simulink model "SADproject"  (R2022b)
settings: Solver=ode5  StartTime=0.0  StopTime=Tsc  FixedStep=0.1  MaxStep=0.1  RelTol=1e-6
values from neighbouring files (symbols this model uses):
  a = R_E+altittude    [SCparameters.m]
  A_iw = [-1  1  1 -1 ... (first row only)    [SCparameters.m]
  A_lin = [     zeros(3)       ,        eye(3) ... (first row only)    [SCparameters.m]
  Ai = [A1 A2 A3 A4 A5 A6 A7 A8 A9 A10]    [SCparameters.m]
  Ai_LN = [1    0      0 ... (first row only)    [SCparameters.m]
  ARW_gyro = 0.15    [SCparameters.m]
  B_lin = [zeros(3); diag(1./diag(J))]    [SCparameters.m]
  bias_gyro = 0.3    [SCparameters.m]
  C_lin = [eye(3), zeros(3)]    [SCparameters.m]
  c_m = (R_E^3*H0)/a^3    [SCparameters.m]
  err_HS = 0.1    [SCparameters.m]
  err_SS = 0.1    [SCparameters.m]
  Fe_E = 117    [SCparameters.m]
  Fe_reflected = 500    [SCparameters.m]
  Fe_Sun = astroConstants(31)    [SCparameters.m]
  i = acos(-(a/12352)^(7/2))    [SCparameters.m]
  i_E = astroConstants(8)    [SCparameters.m]
  i_m = deg2rad(11.5)    [SCparameters.m]
  J = I_body + I_panel1 + I_panel2    [SCparameters.m]
  L = place(A_lin',C_lin',CLP)'    [SCparameters.m]
  m = [0.01 0.05 0.01]'    [SCparameters.m]
  maxL_iw = 6*1e-3    (= 0.006)    [SCparameters.m]
  maxT_iw = 0.1*1e-3    (= 0.0001)    [SCparameters.m]
  n = sqrt(muE/a^3)    [SCparameters.m]
  N_Bi = [n1; n2; n3; n4; n5; n6; n7; n8; n9; n10]    [SCparameters.m]
  n_Sun = 2*pi/T_E    (= 1.99098857148e-07)    [SCparameters.m]
  om0 = [1 1 1]'    [SCparameters.m]
  om_E = 7.292*1e-5    (= 7.292e-05)    [SCparameters.m]
  pinvA_iw = [-1 -1  1 ... (first row only)    [SCparameters.m]
  R_t = [R_t1; R_t2]    [SCparameters.m]
  Ri = [b0; b0; b0; b0; b0; b0; b1; b1; b2; b2]    [SCparameters.m]
  T = 0.005    [SCparameters.m]
undefined symbols (not defined in the file or in its folder): K
libraries: vrlib x13, matrix_library x8, dspinverses x2, simulink_extras x2, sharedutil x2, aerolibutil x1
settings Model: Creator=franc  LastModifiedBy=franc
settings SolverCC: AlgebraicLoopSolver=TrustRegion
settings DebuggingCC: UnconnectedInputMsg=warning  UnconnectedOutputMsg=warning  UnconnectedLineMsg=warning  SFMachineParentedDataDiag=warning
settings ModelReferenceCC: EnableRefExpFcnMdlSchedulingChecks=on

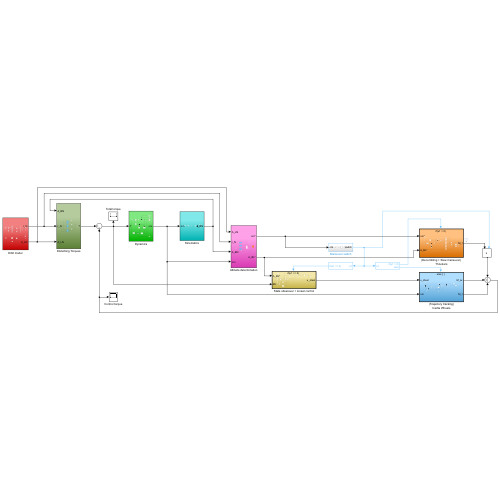
[thumbnail: Simulink's stored preview of the top-level diagram]
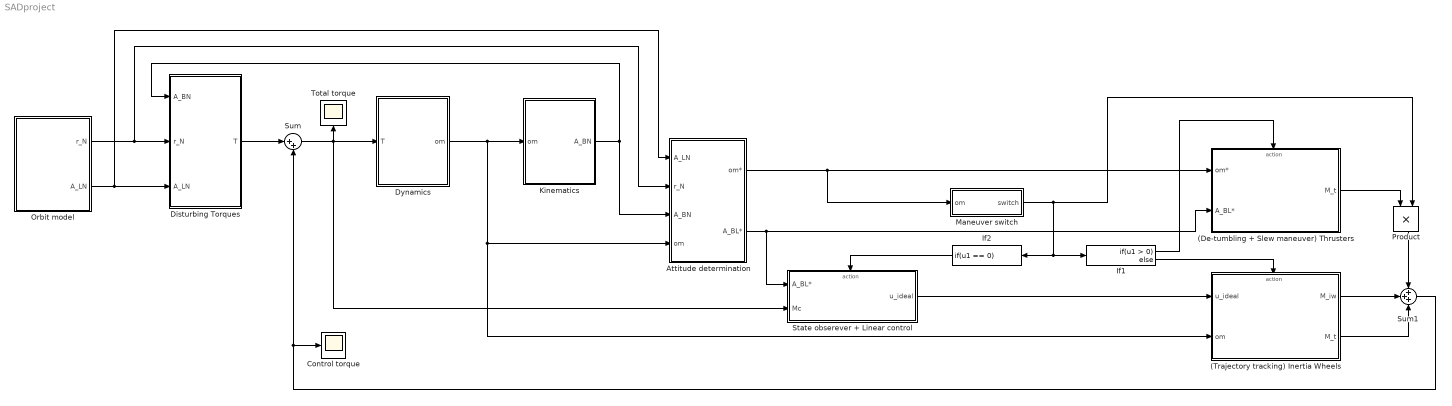
== system SADproject ==
  (De-tumbling + Slew maneuver) Thrusters : Subsystem  TreatAsAtomicUnit=on
  (Trajectory tracking) Inertia Wheels : Subsystem  TreatAsAtomicUnit=on
  Attitude determination : Subsystem
  Control torque : Scope
  Disturbing Torques : Subsystem
  Dynamics : Subsystem
  If1 : If
  If2 : If  IfExpression=u1 == 0  ShowElse=off
  Kinematics : Subsystem
  Maneuver switch : Subsystem
  "Orbit model " : Subsystem
  Product : Product
  State obserever + Linear control : Subsystem
  Sum : Sum  Inputs=|++
  Sum1 : Sum  Inputs=+++
  Total torque : Scope
  wires:
  (De-tumbling + Slew maneuver) Thrusters/1(M_t) -> Product/1
  (Trajectory tracking) Inertia Wheels/1(M_iw) -> Sum1/2
  Product/1 -> Sum1/1
  (Trajectory tracking) Inertia Wheels/2(M_t) -> Sum1/3
  Sum1/1 -> Sum/2, Control torque/1
  State obserever + Linear control/1(u_ideal) -> (Trajectory tracking) Inertia Wheels/1(u_ideal)
  Sum/1 -> State obserever + Linear control/2(Mc), Dynamics/1(T), Total torque/1
  Maneuver switch/1(switch) -> If2/1, If1/1, Product/2
  If1/1 -> (De-tumbling + Slew maneuver) Thrusters/Action
  If1/2 -> (Trajectory tracking) Inertia Wheels/Action
  If2/1 -> State obserever + Linear control/Action
  Dynamics/1(om) -> Kinematics/1(om), (Trajectory tracking) Inertia Wheels/2(om), Attitude determination/4(om)
  Attitude determination/2(A_BL*) -> State obserever + Linear control/1(A_BL*), (De-tumbling + Slew maneuver) Thrusters/2(A_BL*)
  Attitude determination/1(om*) -> (De-tumbling + Slew maneuver) Thrusters/1(om*), Maneuver switch/1(om)
  Kinematics/1(A_BN) -> Attitude determination/3(A_BN), Disturbing Torques/1(A_BN)
  "Orbit model "/1(r_N) -> Disturbing Torques/2(r_N), Attitude determination/2(r_N)
  "Orbit model "/2(A_LN) -> Disturbing Torques/3(A_LN), Attitude determination/1(A_LN)
  Disturbing Torques/1(T) -> Sum/1

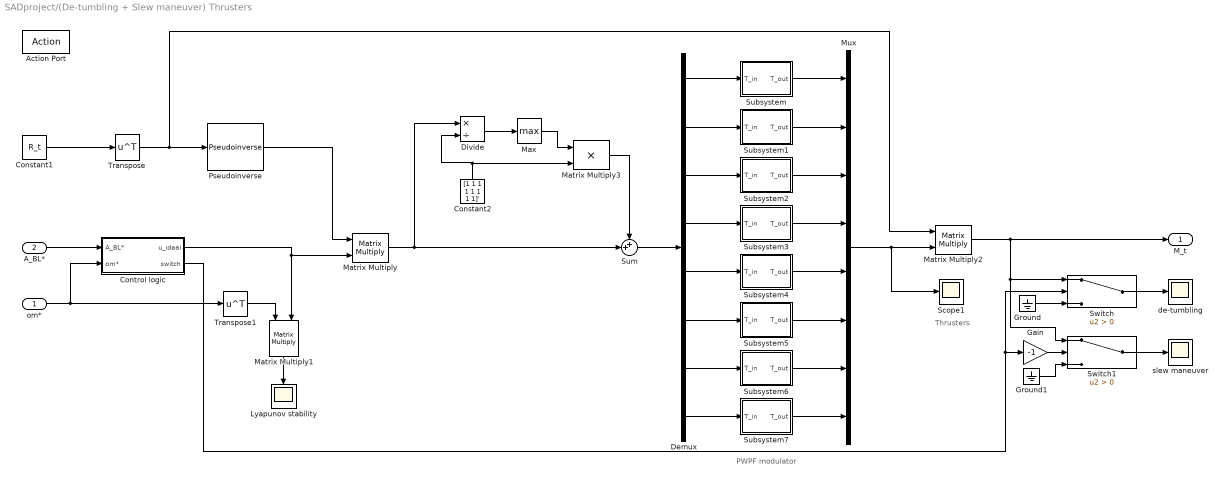
== system SADproject/(De-tumbling + Slew maneuver) Thrusters ==
  note: Thrusters
  note: PWPF modulator
  om* : Inport
  A_BL* : Inport  Port=2
  Action Port : ActionPort  ActionPortLabel=if(u1 > 0)
  Constant1 : Constant  Value=R_t
  Constant2 : Constant  Value=[1 1 1 1 1 1 1 1]'
  Control logic : Subsystem
  Demux : Demux  Outputs=8
  Divide : Product  Inputs=*/
  Gain : Gain  Gain=-1
  Ground : Ground
  Ground1 : Ground
  Lyapunov stability : Scope
  Matrix Multiply : Product  Multiplication=Matrix(*)
  Matrix Multiply1 : Product  Multiplication=Matrix(*)
  Matrix Multiply2 : Product  Multiplication=Matrix(*)
  Matrix Multiply3 : Product
  Max : MinMax  Function=max
  Mux : Mux  Inputs=8
  Pseudoinverse : dspinverses/Pseudoinverse  wanterr=off  SimulateUsing=Interpreted execution
  Scope1 : Scope
  Subsystem : Subsystem
  Subsystem1 : Subsystem
  Subsystem2 : Subsystem
  Subsystem3 : Subsystem
  Subsystem4 : Subsystem
  Subsystem5 : Subsystem
  Subsystem6 : Subsystem
  Subsystem7 : Subsystem
  Sum : Sum  Inputs=++|
  Switch : Switch  Criteria=u2 > Threshold  SaturateOnIntegerOverflow=off  InputSameDT=off
  Switch1 : Switch  Criteria=u2 > Threshold  SaturateOnIntegerOverflow=off  InputSameDT=off
  Transpose : Math  Operator=transpose
  Transpose1 : Math  Operator=transpose
  de-tumbling : Scope
  slew maneuver : Scope
  M_t : Outport
  wires:
  Subsystem1/1(T_out) -> Mux/2
  Demux/8 -> Subsystem7/1(T_in)
  Demux/7 -> Subsystem6/1(T_in)
  Subsystem2/1(T_out) -> Mux/3
  Subsystem7/1(T_out) -> Mux/8
  Demux/4 -> Subsystem3/1(T_in)
  Subsystem3/1(T_out) -> Mux/4
  Demux/6 -> Subsystem5/1(T_in)
  Demux/2 -> Subsystem1/1(T_in)
  Demux/3 -> Subsystem2/1(T_in)
  Constant2/1 -> Matrix Multiply3/2, Divide/2
  Subsystem5/1(T_out) -> Mux/6
  Matrix Multiply1/1 -> Lyapunov stability/1
  Matrix Multiply2/1 -> Switch1/1, Switch/1, M_t/1
  Subsystem/1(T_out) -> Mux/1
  Mux/1 -> Scope1/1, Matrix Multiply2/2
  Matrix Multiply3/1 -> Sum/1
  om*/1 -> Control logic/2(om*), Transpose1/1
  Subsystem6/1(T_out) -> Mux/7
  Pseudoinverse/1 -> Matrix Multiply/1
  Divide/1 -> Max/1
  Matrix Multiply/1 -> Sum/2, Divide/1
  Max/1 -> Matrix Multiply3/1
  Constant1/1 -> Transpose/1
  Transpose/1 -> Matrix Multiply2/1, Pseudoinverse/1
  Demux/1 -> Subsystem/1(T_in)
  Control logic/1(u_ideal) -> Matrix Multiply/2, Matrix Multiply1/2
  Demux/5 -> Subsystem4/1(T_in)
  Sum/1 -> Demux/1
  Subsystem4/1(T_out) -> Mux/5
  Transpose1/1 -> Matrix Multiply1/1
  A_BL*/1 -> Control logic/1(A_BL*)
  Control logic/2(switch) -> Switch/2, Gain/1
  Ground/1 -> Switch/3
  Switch/1 -> de-tumbling/1
  Gain/1 -> Switch1/2
  Ground1/1 -> Switch1/3
  Switch1/1 -> slew maneuver/1

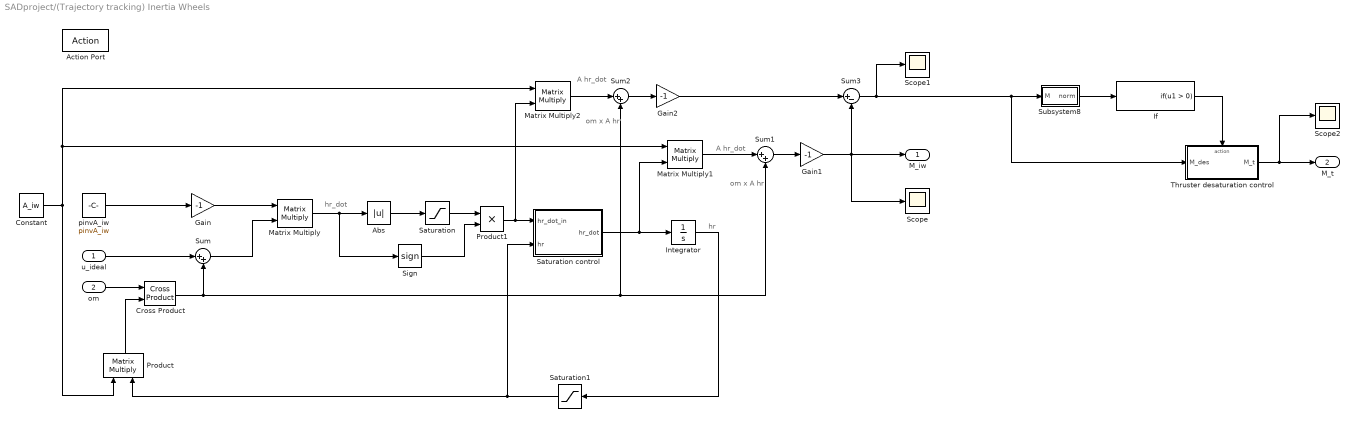
== system SADproject/(Trajectory tracking) Inertia Wheels ==
  note: hr_dot
  note: hr
  note: om x A hr
  note: A hr_dot
  note: A hr_dot
  note: om x A hr
  u_ideal : Inport
  om : Inport  Port=2
  Action Port : ActionPort  ActionPortLabel=else
  Abs : Abs  SaturateOnIntegerOverflow=off
  Constant : Constant  Value=A_iw
  Cross Product : matrix_library/Cross Product
  Gain : Gain  Gain=-1
  Gain1 : Gain  Gain=-1
  Gain2 : Gain  Gain=-1
  If : If  ShowElse=off
  Integrator : Integrator  InitialCondition=[0 0 0 0]
  Matrix Multiply : Product  Multiplication=Matrix(*)
  Matrix Multiply1 : Product  Multiplication=Matrix(*)
  Matrix Multiply2 : Product  Multiplication=Matrix(*)
  Product : Product  Multiplication=Matrix(*)
  Product1 : Product
  Saturation : Saturate  UpperLimit=maxT_iw  LowerLimit=0
  Saturation control : Subsystem
  Saturation1 : Saturate  UpperLimit=maxL_iw  LowerLimit=-maxL_iw
  Scope : Scope
  Scope1 : Scope
  Scope2 : Scope
  Sign : Signum
  Subsystem8 : Subsystem
  Sum : Sum  Inputs=|++
  Sum1 : Sum  Inputs=|++
  Sum2 : Sum  Inputs=|++
  Sum3 : Sum  Inputs=|+-
  Thruster desaturation control : Subsystem
  pinvA_iw : Constant  Value=pinvA_iw
  M_iw : Outport
  M_t : Outport  Port=2
  wires:
  Sum3/1 -> Thruster desaturation control/1(M_des), Subsystem8/1(M), Scope1/1
  If/1 -> Thruster desaturation control/Action
  Thruster desaturation control/1(M_t) -> Scope2/1, M_t/1
  Subsystem8/1(norm) -> If/1
  Product/1 -> Cross Product/2
  Sum/1 -> Matrix Multiply/2
  om/1 -> Cross Product/1
  Product1/1 -> Matrix Multiply2/2, Saturation control/1(hr_dot_in)
  Gain1/1 -> Sum3/2, Scope/1, M_iw/1
  Gain2/1 -> Sum3/1
  Integrator/1 -> Saturation1/1
  Matrix Multiply2/1 -> Sum2/1
  Matrix Multiply1/1 -> Sum1/1
  Gain/1 -> Matrix Multiply/1
  Sign/1 -> Product1/2
  Cross Product/1 -> Sum2/2, Sum1/2, Sum/2
  Saturation1/1 -> Product/2, Saturation control/2(hr)
  Sum1/1 -> Gain1/1
  Constant/1 -> Product/1, Matrix Multiply2/1, Matrix Multiply1/1
  Matrix Multiply/1 -> Sign/1, Abs/1
  Saturation/1 -> Product1/1
  Sum2/1 -> Gain2/1
  pinvA_iw/1 -> Gain/1
  Saturation control/1(hr_dot) -> Matrix Multiply1/2, Integrator/1
  u_ideal/1 -> Sum/1
  Abs/1 -> Saturation/1

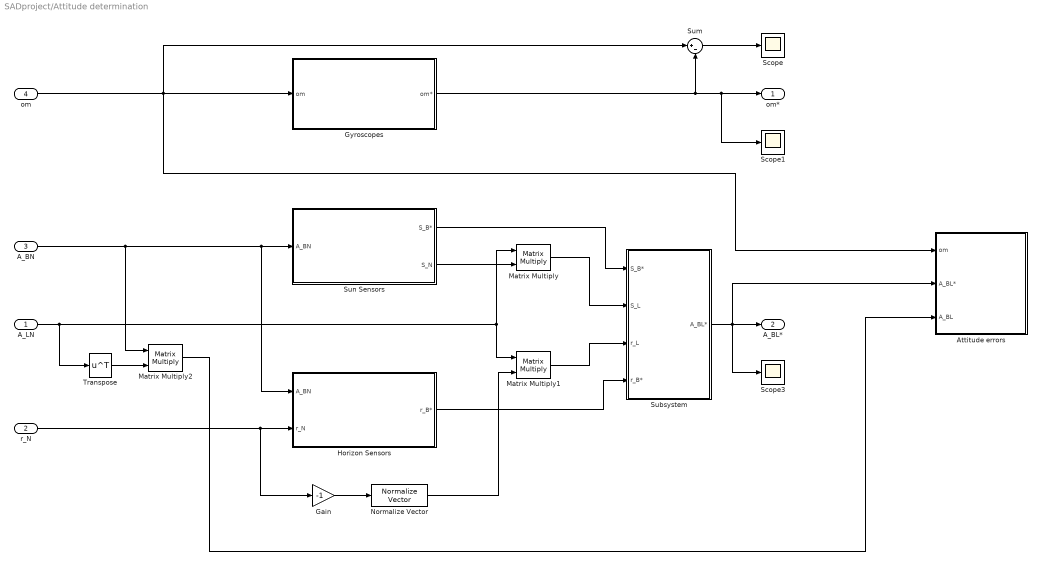
== system SADproject/Attitude determination ==
  A_LN : Inport
  r_N : Inport  Port=2
  A_BN : Inport  Port=3
  om : Inport  Port=4
  Attitude errors : Subsystem
  Gain : Gain  Gain=-1
  Gyroscopes : Subsystem
  Horizon Sensors : Subsystem
  Matrix Multiply : Product  Multiplication=Matrix(*)
  Matrix Multiply1 : Product  Multiplication=Matrix(*)
  Matrix Multiply2 : Product  Multiplication=Matrix(*)
  Normalize Vector : vrlib/Utilities/Normalize Vector  maxzero=0
  Scope : Scope
  Scope1 : Scope
  Scope3 : Scope
  Subsystem : Subsystem
  Sum : Sum  Inputs=|+-
  Sun Sensors : Subsystem
  Transpose : Math  Operator=transpose
  om* : Outport
  A_BL* : Outport  Port=2
  wires:
  om/1 -> Attitude errors/1(om), Sum/1, Gyroscopes/1(om)
  Gyroscopes/1("om* ") -> Sum/2, Scope1/1, om*/1
  A_BN/1 -> Matrix Multiply2/1, Horizon Sensors/1(A_BN), Sun Sensors/1(A_BN)
  r_N/1 -> Gain/1, Horizon Sensors/2(r_N)
  Sun Sensors/2(S_N) -> Matrix Multiply/2
  A_LN/1 -> Transpose/1, Matrix Multiply1/1, Matrix Multiply/1
  Gain/1 -> Normalize Vector/1
  Normalize Vector/1 -> Matrix Multiply1/2
  Matrix Multiply1/1 -> Subsystem/3(r_L)
  Matrix Multiply/1 -> Subsystem/2(S_L)
  Sun Sensors/1(S_B*) -> Subsystem/1(S_B*)
  Horizon Sensors/1(r_B*) -> Subsystem/4(r_B*)
  Subsystem/1(A_BL*) -> Scope3/1, Attitude errors/2(A_BL*), A_BL*/1
  Transpose/1 -> Matrix Multiply2/2
  Matrix Multiply2/1 -> Attitude errors/3(A_BL)
  Sum/1 -> Scope/1

== system SADproject/Disturbing Torques ==
  A_BN : Inport
  r_N : Inport  Port=2
  A_LN : Inport  Port=3
  GG : Scope
  Gravity Gradient : Subsystem
  M : Scope
  Magnetic perturbation : Subsystem
  SRP : Scope
  SRP perturbation : Subsystem
  Scope3 : Scope
  Sum : Sum  Inputs=+++
  T : Outport
  wires:
  r_N/1 -> SRP perturbation/2(r_N), Magnetic perturbation/2(r_N)
  A_BN/1 -> Gravity Gradient/1(A_BN), Magnetic perturbation/1(A_BN), SRP perturbation/1(A_BN)
  SRP perturbation/1(T_SRP) -> SRP/1, Sum/2
  Magnetic perturbation/1(M) -> M/1, Sum/3
  Gravity Gradient/1(GG) -> GG/1, Sum/1
  Sum/1 -> T/1, Scope3/1
  A_LN/1 -> Gravity Gradient/2(A_LN)

== system SADproject/Dynamics ==
  note: om
  note: om'
  T : Inport
  " " : Constant  Value=J
  Cross Product : matrix_library/Cross Product
  Integrator1 : Integrator  InitialCondition=om0
  Invert 3x3 Matrix : aerolibutil/Invert  3x3 Matrix
  Product1 : Product  Multiplication=Matrix(*)
  Product3 : Product  Multiplication=Matrix(*)
  Scope1 : Scope
  Sum : Sum  Inputs=|++
  To Workspace : ToWorkspace  VariableName=om  SaveFormat=Timeseries  SampleTime=-1
  om : Outport
  wires:
  " "/1 -> Product3/1, Invert 3x3 Matrix/1
  Invert 3x3 Matrix/1 -> Product1/1
  Integrator1/1 -> To Workspace/1, om/1, Product3/2, Cross Product/2, Scope1/1
  Product3/1 -> Cross Product/1
  Sum/1 -> Product1/2
  Product1/1 -> Integrator1/1
  Cross Product/1 -> Sum/1
  T/1 -> Sum/2

== system SADproject/Kinematics ==
  note: A
  note: A'
  om : Inport
  Determinant of 3x3 Matrix : sharedutil/Determinant of 3x3 Matrix  aMode=aMode
  Gain3 : Gain  Gain=-1
  Integrator : Integrator  InitialCondition=eye(3)
  MatrixMultiply : Product  Multiplication=Matrix(*)
  Orthonormalization : Subsystem
  Scope : Scope
  Scope1 : Scope
  To Workspace : ToWorkspace  VariableName=A_BN  SaveFormat=Timeseries  SampleTime=-1
  om^ : Subsystem
  A_BN : Outport
  wires:
  Integrator/1 -> MatrixMultiply/2, Orthonormalization/1(In1)
  MatrixMultiply/1 -> Integrator/1
  Gain3/1 -> MatrixMultiply/1
  Determinant of 3x3 Matrix/1 -> Scope/1
  om/1 -> om^/1(In1)
  om^/1(Out1) -> Gain3/1
  Orthonormalization/1(Out1) -> Determinant of 3x3 Matrix/1, Scope1/1, To Workspace/1, A_BN/1

== system SADproject/Maneuver switch ==
  om : Inport
  Exp : Math  Operator=reciprocal
  Relay : Relay  OnSwitchValue=100  OffSwitchValue=0  OnOutputValue=0  OffOutputValue=1
  Subsystem8 : Subsystem
  switch : Outport
  wires:
  Exp/1 -> Relay/1
  Subsystem8/1(norm) -> Exp/1
  om/1 -> Subsystem8/1(om)
  Relay/1 -> switch/1

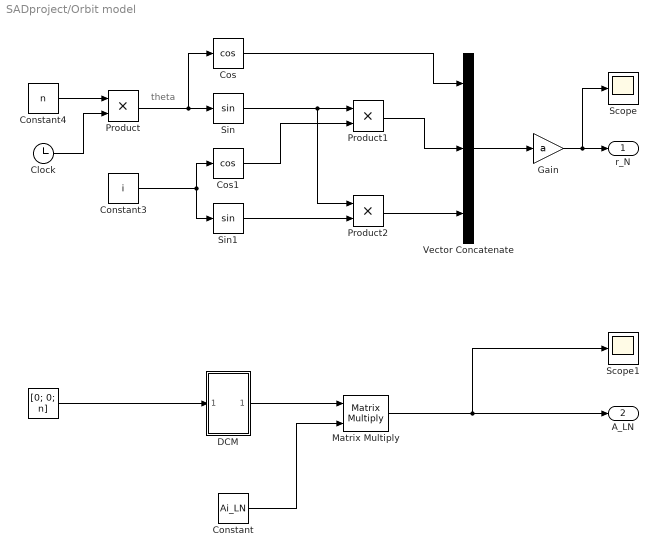
== system SADproject/Orbit model  ==
  note: theta
  " " : Constant  Value=[0; 0; n]
  Clock : Clock
  Constant : Constant  Value=Ai_LN
  Constant3 : Constant  Value=i
  Constant4 : Constant  Value=n
  Cos : Trigonometry  Operator=cos
  Cos1 : Trigonometry  Operator=cos
  DCM : Subsystem
  Gain : Gain  Gain=a
  Matrix Multiply : Product  Multiplication=Matrix(*)
  Product : Product
  Product1 : Product
  Product2 : Product
  Scope : Scope
  Scope1 : Scope
  Sin : Trigonometry
  Sin1 : Trigonometry
  Vector Concatenate : Concatenate  NumInputs=3
  r_N : Outport
  A_LN : Outport  Port=2
  wires:
  Gain/1 -> Scope/1, r_N/1
  Vector Concatenate/1 -> Gain/1
  Product/1 -> Cos/1, Sin/1
  Sin1/1 -> Product2/2
  Product1/1 -> Vector Concatenate/2
  Product2/1 -> Vector Concatenate/3
  Sin/1 -> Product2/1, Product1/1
  Cos/1 -> Vector Concatenate/1
  Clock/1 -> Product/2
  Cos1/1 -> Product1/2
  Constant3/1 -> Sin1/1, Cos1/1
  Constant4/1 -> Product/1
  Matrix Multiply/1 -> Scope1/1, A_LN/1
  DCM/1(A_LN) -> Matrix Multiply/1
  " "/1 -> DCM/1(In1)
  Constant/1 -> Matrix Multiply/2

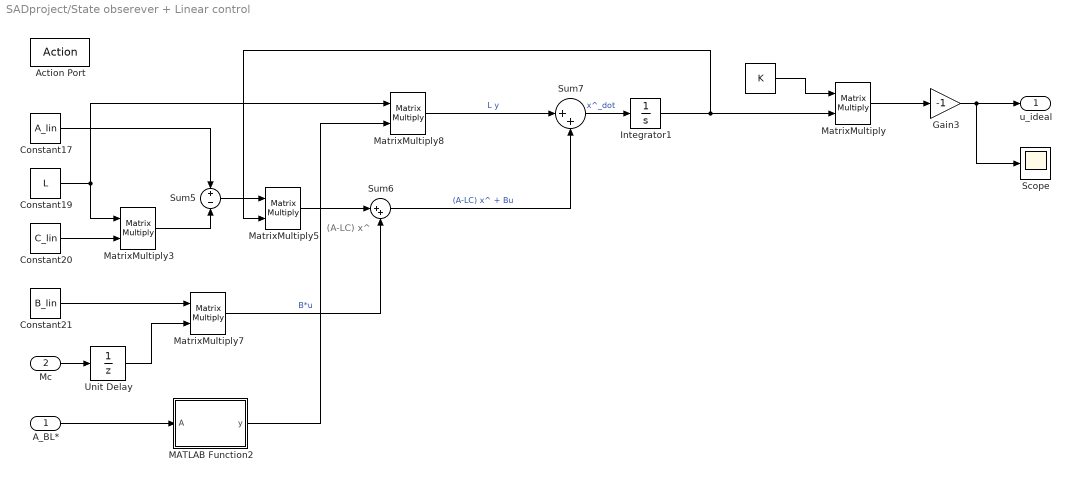
== system SADproject/State obserever + Linear control ==
  note: (A-LC) x^
  A_BL* : Inport
  Mc : Inport  Port=2
  Action Port : ActionPort  ActionPortLabel=if(u1 == 0)
  " " : Constant  Value=K
  Constant17 : Constant  Value=A_lin
  Constant19 : Constant  Value=L
  Constant20 : Constant  Value=C_lin
  Constant21 : Constant  Value=B_lin
  Gain3 : Gain  Gain=-1
  Integrator1 : Integrator  InitialCondition=[0;0;0;0;0;0]
  MATLAB Function2 : MATLAB Function  TreatAsAtomicUnit=on
  MatrixMultiply{,3,5,7..8} (5 alike) : Product  Multiplication=Matrix(*)
  Scope : Scope
  Sum5 : Sum  Inputs=+-
  Sum6 : Sum  Inputs=|++
  Sum7 : Sum  Inputs=|++
  Unit Delay : UnitDelay  SampleTime=-1  HasFrameUpgradeWarning=on
  u_ideal : Outport
  wires:
  Constant17/1 -> Sum5/1
  Sum7/1 -> Integrator1/1  "x^_dot"
  Constant19/1 -> MatrixMultiply3/1, MatrixMultiply8/1
  MatrixMultiply7/1 -> Sum6/2  "B*u"
  Constant20/1 -> MatrixMultiply3/2
  MATLAB Function2/1(y) -> MatrixMultiply8/2
  Sum5/1 -> MatrixMultiply5/1
  MatrixMultiply8/1 -> Sum7/1  "L y"
  MatrixMultiply3/1 -> Sum5/2
  Sum6/1 -> Sum7/2  "(A-LC) x^ + Bu"
  MatrixMultiply5/1 -> Sum6/1
  Constant21/1 -> MatrixMultiply7/1
  Integrator1/1 -> MatrixMultiply/2, MatrixMultiply5/2
  Mc/1 -> Unit Delay/1
  " "/1 -> MatrixMultiply/1
  Gain3/1 -> Scope/1, u_ideal/1
  MatrixMultiply/1 -> Gain3/1
  A_BL*/1 -> MATLAB Function2/1(A)
  Unit Delay/1 -> MatrixMultiply7/2

== system SADproject/(De-tumbling + Slew maneuver) Thrusters/Control logic ==
  A_BL* : Inport
  om* : Inport  Port=2
  De-tumbling : Subsystem
  Exp : Math  Operator=reciprocal
  Relay : Relay  OnSwitchValue=50  OffSwitchValue=0  OnOutputValue=-1  OffOutputValue=1
  Slew maneuver : Subsystem
  Subsystem8 : Subsystem
  Switch : Switch  Criteria=u2 > Threshold  SaturateOnIntegerOverflow=off  InputSameDT=off
  u_ideal : Outport
  switch : Outport  Port=2
  wires:
  om*/1 -> De-tumbling/1(om), Subsystem8/1(om), Slew maneuver/1(om)
  A_BL*/1 -> Slew maneuver/2(A_BL*)
  De-tumbling/1(u_ideal) -> Switch/1
  Slew maneuver/1(u_ideal) -> Switch/3
  Switch/1 -> u_ideal/1
  Subsystem8/1(norm) -> Exp/1
  Exp/1 -> Relay/1
  Relay/1 -> switch/1, Switch/2

== system SADproject/(De-tumbling + Slew maneuver) Thrusters/Subsystem ==
  T_in : Inport
  Relay : Relay  OnSwitchValue=T  OffSwitchValue=0.8*T  OnOutputValue=T
  Scope{3..6} (4 alike) : Scope
  Sum1 : Sum  Inputs=|+-
  Transfer Fcn : TransferFcn  Denominator=[0.1 1]
  T_out : Outport
  wires:
  Sum1/1 -> Transfer Fcn/1, Scope5/1
  T_in/1 -> Sum1/1, Scope3/1
  Transfer Fcn/1 -> Scope4/1, Relay/1
  Relay/1 -> T_out/1, Sum1/2, Scope6/1

== system SADproject/(De-tumbling + Slew maneuver) Thrusters/Subsystem1 ==
  T_in : Inport
  Relay : Relay  OnSwitchValue=T  OffSwitchValue=0.8*T  OnOutputValue=T
  Scope{3..6} (4 alike) : Scope
  Sum1 : Sum  Inputs=|+-
  Transfer Fcn : TransferFcn  Denominator=[0.1 1]
  T_out : Outport
  wires:
  Relay/1 -> Scope6/1, Sum1/2, T_out/1
  Transfer Fcn/1 -> Relay/1, Scope4/1
  T_in/1 -> Scope3/1, Sum1/1
  Sum1/1 -> Scope5/1, Transfer Fcn/1

== system SADproject/(De-tumbling + Slew maneuver) Thrusters/Subsystem2 ==
  T_in : Inport
  Relay : Relay  OnSwitchValue=T  OffSwitchValue=0.8*T  OnOutputValue=T
  Scope{3..6} (4 alike) : Scope
  Sum1 : Sum  Inputs=|+-
  Transfer Fcn : TransferFcn  Denominator=[0.1 1]
  T_out : Outport
  wires:
  Sum1/1 -> Transfer Fcn/1, Scope5/1
  T_in/1 -> Sum1/1, Scope3/1
  Transfer Fcn/1 -> Scope4/1, Relay/1
  Relay/1 -> T_out/1, Sum1/2, Scope6/1

== system SADproject/(De-tumbling + Slew maneuver) Thrusters/Subsystem3 ==
  T_in : Inport
  Relay : Relay  OnSwitchValue=T  OffSwitchValue=0.8*T  OnOutputValue=T
  Scope{3..6} (4 alike) : Scope
  Sum1 : Sum  Inputs=|+-
  Transfer Fcn : TransferFcn  Denominator=[0.1 1]
  T_out : Outport
  wires:
  Relay/1 -> Scope6/1, Sum1/2, T_out/1
  Transfer Fcn/1 -> Relay/1, Scope4/1
  T_in/1 -> Scope3/1, Sum1/1
  Sum1/1 -> Scope5/1, Transfer Fcn/1

== system SADproject/(De-tumbling + Slew maneuver) Thrusters/Subsystem4 ==
  T_in : Inport
  Relay : Relay  OnSwitchValue=T  OffSwitchValue=0.8*T  OnOutputValue=T
  Scope{3..6} (4 alike) : Scope
  Sum1 : Sum  Inputs=|+-
  Transfer Fcn : TransferFcn  Denominator=[0.1 1]
  T_out : Outport
  wires:
  Sum1/1 -> Transfer Fcn/1, Scope5/1
  T_in/1 -> Sum1/1, Scope3/1
  Transfer Fcn/1 -> Scope4/1, Relay/1
  Relay/1 -> T_out/1, Sum1/2, Scope6/1

== system SADproject/(De-tumbling + Slew maneuver) Thrusters/Subsystem5 ==
  T_in : Inport
  Relay : Relay  OnSwitchValue=T  OffSwitchValue=0.8*T  OnOutputValue=T
  Scope{3..6} (4 alike) : Scope
  Sum1 : Sum  Inputs=|+-
  Transfer Fcn : TransferFcn  Denominator=[0.1 1]
  T_out : Outport
  wires:
  Relay/1 -> Scope6/1, Sum1/2, T_out/1
  Transfer Fcn/1 -> Relay/1, Scope4/1
  T_in/1 -> Scope3/1, Sum1/1
  Sum1/1 -> Scope5/1, Transfer Fcn/1

== system SADproject/(De-tumbling + Slew maneuver) Thrusters/Subsystem6 ==
  T_in : Inport
  Relay : Relay  OnSwitchValue=T  OffSwitchValue=0.8*T  OnOutputValue=T
  Scope{3..6} (4 alike) : Scope
  Sum1 : Sum  Inputs=|+-
  Transfer Fcn : TransferFcn  Denominator=[0.1 1]
  T_out : Outport
  wires:
  Sum1/1 -> Transfer Fcn/1, Scope5/1
  T_in/1 -> Sum1/1, Scope3/1
  Transfer Fcn/1 -> Scope4/1, Relay/1
  Relay/1 -> T_out/1, Sum1/2, Scope6/1

== system SADproject/(De-tumbling + Slew maneuver) Thrusters/Subsystem7 ==
  T_in : Inport
  Relay : Relay  OnSwitchValue=T  OffSwitchValue=0.8*T  OnOutputValue=T
  Scope{3..6} (4 alike) : Scope
  Sum1 : Sum  Inputs=|+-
  Transfer Fcn : TransferFcn  Denominator=[0.1 1]
  T_out : Outport
  wires:
  Relay/1 -> Scope6/1, Sum1/2, T_out/1
  Transfer Fcn/1 -> Relay/1, Scope4/1
  T_in/1 -> Scope3/1, Sum1/1
  Sum1/1 -> Scope5/1, Transfer Fcn/1

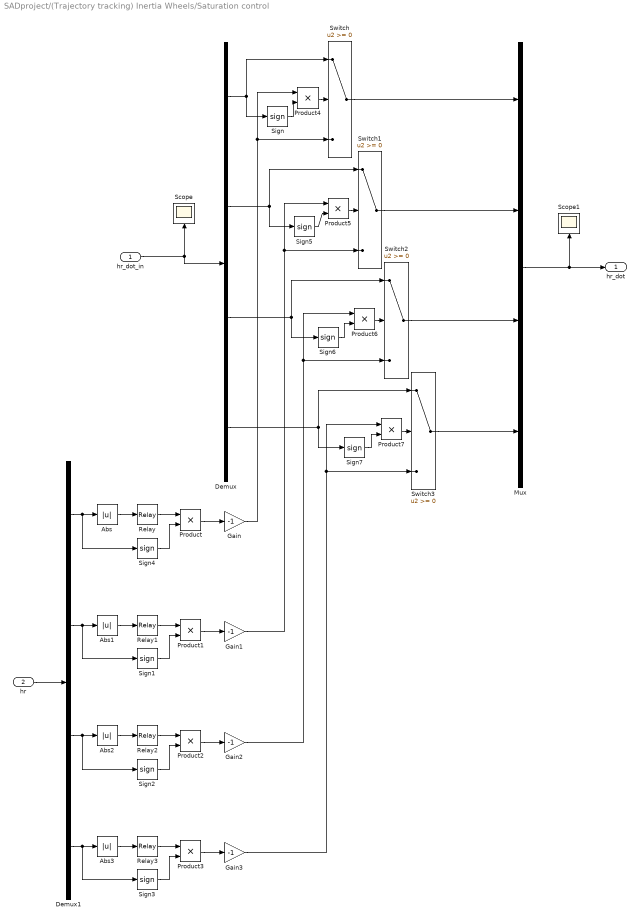
== system SADproject/(Trajectory tracking) Inertia Wheels/Saturation control ==
  hr_dot_in : Inport
  hr : Inport  Port=2
  Abs{,1..3} (4 alike) : Abs  SaturateOnIntegerOverflow=off
  Demux : Demux
  Demux1 : Demux
  Gain{,1..3} (4 alike) : Gain  Gain=-1
  Mux : Mux
  Product{,1..7} (8 alike) : Product
  Relay{,1..3} (4 alike) : Relay  OnSwitchValue=maxL_iw  OffSwitchValue=maxL_iw/1000  OnOutputValue=maxT_iw
  Scope : Scope
  Scope1 : Scope
  Sign{,1..7} (8 alike) : Signum
  Switch{,1..3} (4 alike) : Switch  SaturateOnIntegerOverflow=off  InputSameDT=off
  hr_dot : Outport
  wires:
  hr/1 -> Demux1/1
  hr_dot_in/1 -> Scope/1, Demux/1
  Mux/1 -> Scope1/1, hr_dot/1
  Relay/1 -> Product/1
  Sign4/1 -> Product/2
  Product/1 -> Gain/1
  Abs/1 -> Relay/1
  Demux1/1 -> Sign4/1, Abs/1
  Demux1/2 -> Abs1/1, Sign1/1
  Abs1/1 -> Relay1/1
  Product1/1 -> Gain1/1
  Sign1/1 -> Product1/2
  Relay1/1 -> Product1/1
  Relay2/1 -> Product2/1
  Sign2/1 -> Product2/2
  Product2/1 -> Gain2/1
  Abs2/1 -> Relay2/1
  Demux1/3 -> Sign2/1, Abs2/1
  Demux1/4 -> Abs3/1, Sign3/1
  Abs3/1 -> Relay3/1
  Product3/1 -> Gain3/1
  Sign3/1 -> Product3/2
  Relay3/1 -> Product3/1
  Demux/1 -> Switch/1, Sign/1
  Switch/1 -> Mux/1
  Gain/1 -> Product4/1, Switch/3
  Gain1/1 -> Product5/1, Switch1/3
  Gain2/1 -> Product6/1, Switch2/3
  Gain3/1 -> Product7/1, Switch3/3
  Sign/1 -> Product4/2
  Product4/1 -> Switch/2
  Product5/1 -> Switch1/2
  Sign5/1 -> Product5/2
  Demux/2 -> Switch1/1, Sign5/1
  Switch1/1 -> Mux/2
  Product6/1 -> Switch2/2
  Sign6/1 -> Product6/2
  Demux/3 -> Switch2/1, Sign6/1
  Product7/1 -> Switch3/2
  Sign7/1 -> Product7/2
  Demux/4 -> Switch3/1, Sign7/1
  Switch3/1 -> Mux/4
  Switch2/1 -> Mux/3

== system SADproject/(Trajectory tracking) Inertia Wheels/Subsystem8 ==
  M : Inport
  Dot Product : DotProduct  OutDataTypeStr=Inherit: Inherit via internal rule
  Sqrt : Sqrt
  norm : Outport
  wires:
  Sqrt/1 -> norm/1
  Dot Product/1 -> Sqrt/1
  M/1 -> Dot Product/2, Dot Product/1

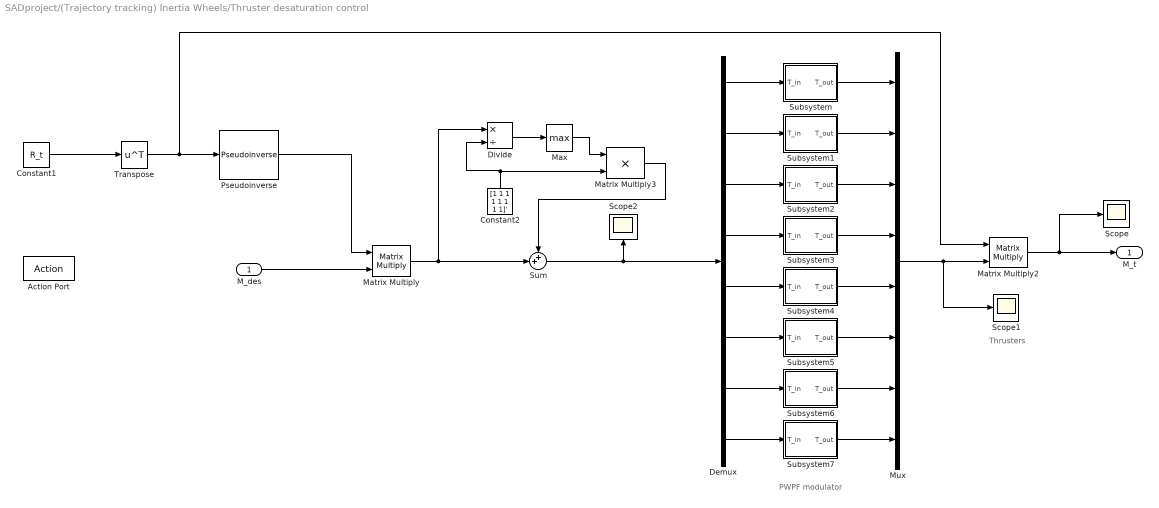
== system SADproject/(Trajectory tracking) Inertia Wheels/Thruster desaturation control ==
  note: Thrusters
  note: PWPF modulator
  M_des : Inport
  Action Port : ActionPort  ActionPortLabel=if(u1 > 0)
  Constant1 : Constant  Value=R_t
  Constant2 : Constant  Value=[1 1 1 1 1 1 1 1]'
  Demux : Demux  Outputs=8
  Divide : Product  Inputs=*/
  Matrix Multiply : Product  Multiplication=Matrix(*)
  Matrix Multiply2 : Product  Multiplication=Matrix(*)
  Matrix Multiply3 : Product
  Max : MinMax  Function=max
  Mux : Mux  Inputs=8
  Pseudoinverse : dspinverses/Pseudoinverse  wanterr=off  SimulateUsing=Interpreted execution
  Scope : Scope
  Scope1 : Scope
  Scope2 : Scope
  Subsystem : Subsystem
  Subsystem1 : Subsystem
  Subsystem2 : Subsystem
  Subsystem3 : Subsystem
  Subsystem4 : Subsystem
  Subsystem5 : Subsystem
  Subsystem6 : Subsystem
  Subsystem7 : Subsystem
  Sum : Sum  Inputs=++|
  Transpose : Math  Operator=transpose
  M_t : Outport
  wires:
  Divide/1 -> Max/1
  Subsystem3/1(T_out) -> Mux/4
  Demux/2 -> Subsystem1/1(T_in)
  Sum/1 -> Demux/1, Scope2/1
  Pseudoinverse/1 -> Matrix Multiply/1
  Subsystem7/1(T_out) -> Mux/8
  Demux/5 -> Subsystem4/1(T_in)
  Matrix Multiply/1 -> Sum/2, Divide/1
  Subsystem4/1(T_out) -> Mux/5
  Transpose/1 -> Matrix Multiply2/1, Pseudoinverse/1
  Demux/7 -> Subsystem6/1(T_in)
  Demux/1 -> Subsystem/1(T_in)
  Subsystem6/1(T_out) -> Mux/7
  Matrix Multiply3/1 -> Sum/1
  Mux/1 -> Scope1/1, Matrix Multiply2/2
  Matrix Multiply2/1 -> M_t/1, Scope/1
  Max/1 -> Matrix Multiply3/1
  Constant1/1 -> Transpose/1
  Constant2/1 -> Matrix Multiply3/2, Divide/2
  Subsystem2/1(T_out) -> Mux/3
  Demux/8 -> Subsystem7/1(T_in)
  Subsystem1/1(T_out) -> Mux/2
  Demux/4 -> Subsystem3/1(T_in)
  Demux/3 -> Subsystem2/1(T_in)
  Demux/6 -> Subsystem5/1(T_in)
  Subsystem/1(T_out) -> Mux/1
  Subsystem5/1(T_out) -> Mux/6
  M_des/1 -> Matrix Multiply/2

== system SADproject/Attitude determination/Attitude errors ==
  om : Inport
  A_BL* : Inport  Port=2
  A_BL : Inport  Port=3
  Measured : Subsystem
  Sum : Sum  Inputs=|+-
  Sum1 : Sum  Inputs=|+-
  True : Subsystem
  alpha_err : Scope
  alphas : Scope
  alphas* : Scope
  om_BL : Scope
  om_BL* : Scope
  om_err : Scope
  wires:
  om/1 -> Measured/1(om), True/2(om)
  A_BL/1 -> True/1(A_BL)
  A_BL*/1 -> Measured/2(A_BL*)
  True/1(alphas) -> Sum/1, alphas/1
  Measured/2(om_BL*) -> Sum1/2, om_BL*/1
  Measured/1(alphas*) -> Sum/2, alphas*/1
  True/2(om_BL) -> Sum1/1, om_BL/1
  Sum/1 -> alpha_err/1
  Sum1/1 -> om_err/1

== system SADproject/Attitude determination/Gyroscopes ==
  om : Inport
  Bias(°/h) : RandomNumber  Mean=[0; 0; 0]  Variance=((deg2rad(bias_gyro))^2)*[1; 1; 1]  Seed=randi(1000, [3, 1])  SampleTime=0.5
  Gain1 : Gain  Gain=1/3600
  Noise : Subsystem
  Scope : Scope
  Sum : Sum  Inputs=+++
  Sum1 : Sum  Inputs=+-
  om_err : Scope
  "om* " : Outport
  wires:
  Sum/1 -> Scope/1, "om* "/1, Sum1/1
  om/1 -> Sum1/2, Sum/2
  Noise/1(Out1) -> Sum/1
  Bias(°/h)/1 -> Gain1/1
  Gain1/1 -> Sum/3
  Sum1/1 -> om_err/1

== system SADproject/Attitude determination/Horizon Sensors ==
  A_BN : Inport
  r_N : Inport  Port=2
  " " : Product  Multiplication=Matrix(*)
  Constant : Constant  Value=[0 1 -1; -1 0 1; 1 -1 0]
  Constant1 : Constant  Value=[1 0 0; 0 1 0; 0 0 1]
  Gain : Gain  Gain=-1
  Matrix Multiply : Product  Multiplication=Matrix(*)
  Normalize Vector : vrlib/Utilities/Normalize Vector  maxzero=0
  Product : Product
  Random Number : RandomNumber  Variance=(deg2rad(err_HS/3))^2  SampleTime=0.5
  Scope : Scope
  Sum : Sum  Inputs=|++
  r_B* : Outport
  wires:
  Matrix Multiply/1 -> Normalize Vector/1
  Sum/1 -> " "/1
  A_BN/1 -> Matrix Multiply/1
  " "/1 -> r_B*/1, Scope/1
  Constant/1 -> Product/2
  Constant1/1 -> Sum/2
  Product/1 -> Sum/1
  Random Number/1 -> Product/1
  Normalize Vector/1 -> " "/2
  r_N/1 -> Gain/1
  Gain/1 -> Matrix Multiply/2

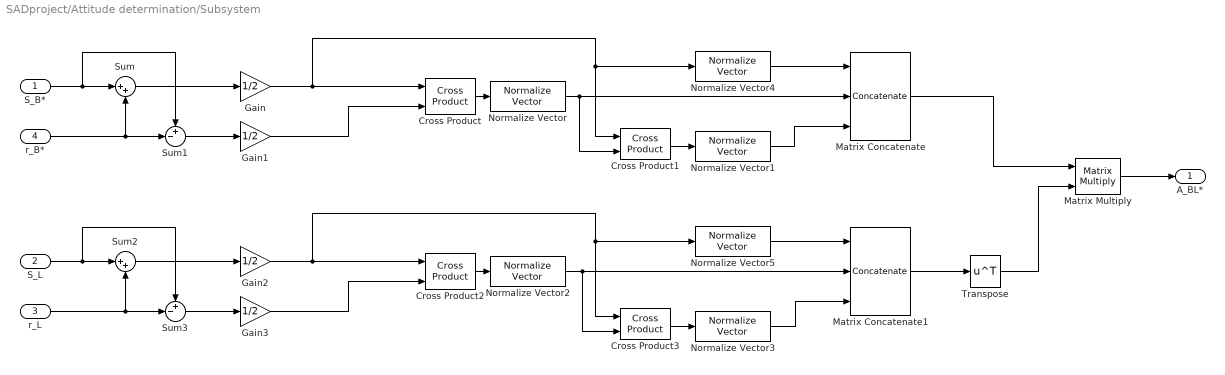
== system SADproject/Attitude determination/Subsystem ==
  S_B* : Inport
  S_L : Inport  Port=2
  r_L : Inport  Port=3
  r_B* : Inport  Port=4
  Cross Product{,1..3} (4 alike) : matrix_library/Cross Product
  Gain{,1..3} (4 alike) : Gain  Gain=1/2
  Matrix Concatenate : Concatenate  NumInputs=3  Mode=Multidimensional array  ConcatenateDimension=2
  Matrix Concatenate1 : Concatenate  NumInputs=3  Mode=Multidimensional array  ConcatenateDimension=2
  Matrix Multiply : Product  Multiplication=Matrix(*)
  Normalize Vector{,1..5} (6 alike) : vrlib/Utilities/Normalize Vector  maxzero=0
  Sum : Sum  Inputs=|++
  Sum1 : Sum  Inputs=+-|
  Sum2 : Sum  Inputs=|++
  Sum3 : Sum  Inputs=+-|
  Transpose : Math  Operator=transpose
  A_BL* : Outport
  wires:
  r_B*/1 -> Sum1/2, Sum/2
  Cross Product1/1 -> Normalize Vector1/1
  Normalize Vector2/1 -> Cross Product3/2, Matrix Concatenate1/2
  Cross Product3/1 -> Normalize Vector3/1
  Cross Product2/1 -> Normalize Vector2/1
  Matrix Concatenate1/1 -> Transpose/1
  Matrix Concatenate/1 -> Matrix Multiply/1
  Transpose/1 -> Matrix Multiply/2
  Matrix Multiply/1 -> A_BL*/1
  Cross Product/1 -> Normalize Vector/1
  Normalize Vector/1 -> Cross Product1/2, Matrix Concatenate/2
  Normalize Vector1/1 -> Matrix Concatenate/3
  Normalize Vector3/1 -> Matrix Concatenate1/3
  S_B*/1 -> Sum1/1, Sum/1
  Sum/1 -> Gain/1
  Gain/1 -> Normalize Vector4/1, Cross Product1/1, Cross Product/1
  Sum1/1 -> Gain1/1
  Gain1/1 -> Cross Product/2
  Normalize Vector4/1 -> Matrix Concatenate/1
  Normalize Vector5/1 -> Matrix Concatenate1/1
  Sum2/1 -> Gain2/1
  r_L/1 -> Sum3/2, Sum2/2
  Gain2/1 -> Cross Product2/1, Cross Product3/1, Normalize Vector5/1
  S_L/1 -> Sum3/1, Sum2/1
  Sum3/1 -> Gain3/1
  Gain3/1 -> Cross Product2/2

== system SADproject/Attitude determination/Sun Sensors ==
  A_BN : Inport
  " " : Product  Multiplication=Matrix(*)
  Constant : Constant  Value=[0 1 -1; -1 0 1; 1 -1 0]
  Constant1 : Constant  Value=[1 0 0; 0 1 0; 0 0 1]
  Product : Product
  Random Number : RandomNumber  Variance=(deg2rad(err_SS/3))^2  SampleTime=0.5
  S_B : Subsystem
  Scope : Scope
  Sum : Sum  Inputs=|++
  S_B* : Outport
  S_N : Outport  Port=2
  wires:
  S_B/1(S_B) -> " "/2
  " "/1 -> S_B*/1, Scope/1
  Sum/1 -> " "/1
  A_BN/1 -> S_B/1(A_BN)
  Product/1 -> Sum/1
  Constant1/1 -> Sum/2
  Constant/1 -> Product/2
  Random Number/1 -> Product/1
  S_B/2(S_N) -> S_N/1

== system SADproject/Disturbing Torques/Gravity Gradient ==
  note: A_BL
  A_BN : Inport
  A_LN : Inport  Port=2
  Constant : Constant  Value=[1; 0; 0]
  Constant1 : Constant  Value=J
  Cross Product : matrix_library/Cross Product
  Gain : Gain  Gain=-3*n^2
  Matrix Multiply : Product  Multiplication=Matrix(*)
  Matrix Multiply2 : Product  Multiplication=Matrix(*)
  Matrix Multiply3 : Product  Multiplication=Matrix(*)
  Scope2 : Scope
  Transpose : Math  Operator=transpose
  GG : Outport
  wires:
  Matrix Multiply2/1 -> Matrix Multiply3/2, Cross Product/2
  Gain/1 -> GG/1, Scope2/1
  Cross Product/1 -> Gain/1
  Matrix Multiply3/1 -> Cross Product/1
  Constant/1 -> Matrix Multiply2/2
  Matrix Multiply/1 -> Matrix Multiply2/1
  Constant1/1 -> Matrix Multiply3/1
  A_LN/1 -> Transpose/1
  Transpose/1 -> Matrix Multiply/2
  A_BN/1 -> Matrix Multiply/1

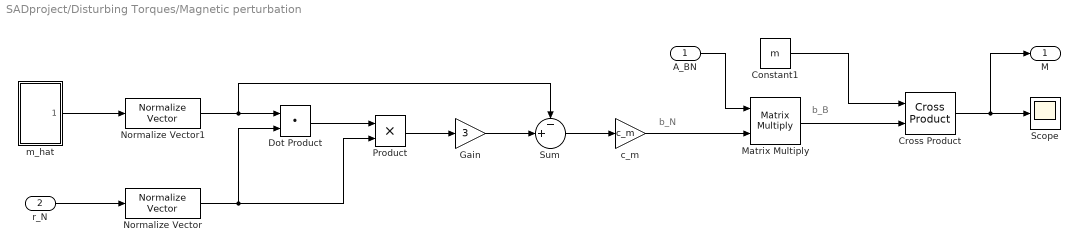
== system SADproject/Disturbing Torques/Magnetic perturbation ==
  note: b_B
  note: b_N
  A_BN : Inport
  r_N : Inport  Port=2
  Constant1 : Constant  Value=m
  Cross Product : matrix_library/Cross Product
  Dot Product : DotProduct  OutDataTypeStr=Inherit: Inherit via internal rule
  Gain : Gain  Gain=3
  Matrix Multiply : Product  Multiplication=Matrix(*)
  Normalize Vector : vrlib/Utilities/Normalize Vector  maxzero=0
  Normalize Vector1 : vrlib/Utilities/Normalize Vector  maxzero=0
  Product : Product
  Scope : Scope
  Sum : Sum  Inputs=-+|
  c_m : Gain  Gain=c_m
  m_hat : Subsystem
  M : Outport
  wires:
  Product/1 -> Gain/1
  c_m/1 -> Matrix Multiply/2
  Normalize Vector/1 -> Product/2, Dot Product/2
  Normalize Vector1/1 -> Sum/1, Dot Product/1
  m_hat/1(m_hat) -> Normalize Vector1/1
  Dot Product/1 -> Product/1
  Matrix Multiply/1 -> Cross Product/2
  Sum/1 -> c_m/1
  Cross Product/1 -> M/1, Scope/1
  r_N/1 -> Normalize Vector/1
  Gain/1 -> Sum/2
  Constant1/1 -> Cross Product/1
  A_BN/1 -> Matrix Multiply/1

== system SADproject/Disturbing Torques/SRP perturbation ==
  note: r_B
  A_BN : Inport
  r_N : Inport  Port=2
  Direct Solar Radiaton : Subsystem
  Earth Radiation : Subsystem
  Gain : Gain  Gain=-1
  Matrix Multiply : Product  Multiplication=Matrix(*)
  Normalize Vector : vrlib/Utilities/Normalize Vector  maxzero=0
  Reflected Radiation : Subsystem
  Scope{,1..3} (4 alike) : Scope
  Sum : Sum  Inputs=+++
  T_SRP : Outport
  wires:
  A_BN/1 -> Direct Solar Radiaton/1(A_BN), Matrix Multiply/1
  Direct Solar Radiaton/1(T_SRP0) -> Scope1/1, Sum/1
  r_N/1 -> Normalize Vector/1
  Matrix Multiply/1 -> Reflected Radiation/1(r_B), Earth Radiation/1(r_B)
  Earth Radiation/1(T_SRP1) -> Scope2/1, Sum/2
  Reflected Radiation/1(T_SRP2) -> Scope3/1, Sum/3
  Sum/1 -> T_SRP/1, Scope/1
  Normalize Vector/1 -> Gain/1
  Gain/1 -> Matrix Multiply/2

== system SADproject/Kinematics/Orthonormalization ==
  In1 : Inport
  Gain4 : Gain  Gain=3/2
  Gain5 : Gain  Gain=1/2
  Matri xMultiply2 : Product  Multiplication=Matrix(*)
  MatrixMultiply1 : Product  Multiplication=Matrix(*)
  Sum : Sum  Inputs=|+-
  Transpose : Math  Operator=transpose
  Out1 : Outport
  wires:
  Matri xMultiply2/1 -> Sum/2
  MatrixMultiply1/1 -> Matri xMultiply2/1
  In1/1 -> Gain5/1, Transpose/1, MatrixMultiply1/1, Gain4/1
  Gain4/1 -> Sum/1
  Gain5/1 -> Matri xMultiply2/2
  Transpose/1 -> MatrixMultiply1/2
  Sum/1 -> Out1/1

== system SADproject/Kinematics/om^ ==
  In1 : Inport
  Gain : Gain  Gain=-1
  Ground : Ground
  Matrix Concatenate : Concatenate  NumInputs=3  Mode=Multidimensional array  ConcatenateDimension=2
  Selector : Selector  InputPortWidth=7  IndexOptions=Index vector (dialog)  Indices=[4 3 6]  OutputSizes=1
  Selector1 : Selector  InputPortWidth=7  IndexOptions=Index vector (dialog)  Indices=[7 4 1]  OutputSizes=1
  Selector2 : Selector  InputPortWidth=7  IndexOptions=Index vector (dialog)  Indices=[2 5 4 ]  OutputSizes=1
  Vector Concatenate : Concatenate  NumInputs=3
  Out1 : Outport
  wires:
  Matrix Concatenate/1 -> Out1/1
  Vector Concatenate/1 -> Selector/1, Selector2/1, Selector1/1
  Ground/1 -> Vector Concatenate/2
  Gain/1 -> Vector Concatenate/3
  In1/1 -> Gain/1, Vector Concatenate/1
  Selector1/1 -> Matrix Concatenate/2
  Selector2/1 -> Matrix Concatenate/3
  Selector/1 -> Matrix Concatenate/1

== system SADproject/Maneuver switch/Subsystem8 ==
  om : Inport
  Dot Product : DotProduct  OutDataTypeStr=Inherit: Inherit via internal rule
  Sqrt : Sqrt
  norm : Outport
  wires:
  Sqrt/1 -> norm/1
  Dot Product/1 -> Sqrt/1
  om/1 -> Dot Product/2, Dot Product/1

== system SADproject/Orbit model /DCM ==
  note: A
  note: A'
  note: om
  In1 : Inport
  Determinant of 3x3 Matrix : sharedutil/Determinant of 3x3 Matrix  aMode=aMode
  Gain3 : Gain  Gain=-1
  Integrator : Integrator  InitialCondition=eye(3)
  MatrixMultiply : Product  Multiplication=Matrix(*)
  Orthonormalization : Subsystem
  Scope : Scope
  Scope1 : Scope
  om^ : Subsystem
  A_LN : Outport
  wires:
  Integrator/1 -> MatrixMultiply/2, Orthonormalization/1(In1)
  MatrixMultiply/1 -> Integrator/1
  Gain3/1 -> MatrixMultiply/1
  Determinant of 3x3 Matrix/1 -> Scope/1
  In1/1 -> om^/1(In1)
  om^/1(Out1) -> Gain3/1
  Orthonormalization/1(Out1) -> Determinant of 3x3 Matrix/1, Scope1/1, A_LN/1

== system SADproject/(De-tumbling + Slew maneuver) Thrusters/Control logic/De-tumbling ==
  om : Inport
  Gain : Gain  Gain=-1
  u_ideal : Outport
  wires:
  om/1 -> Gain/1
  Gain/1 -> u_ideal/1

== system SADproject/(De-tumbling + Slew maneuver) Thrusters/Control logic/Slew maneuver ==
  om : Inport
  A_BL* : Inport  Port=2
  Gain : Gain  Gain=-1
  Gain1 : Gain  Gain=-2/3
  MATLAB Function : MATLAB Function  TreatAsAtomicUnit=on
  Sum : Sum  Inputs=|+-
  Sum1 : Sum  Inputs=|++
  Transpose : Math  Operator=transpose
  u_ideal : Outport
  wires:
  om/1 -> Gain/1
  A_BL*/1 -> Sum/2, Transpose/1
  Transpose/1 -> Sum/1
  Sum/1 -> MATLAB Function/1(A)
  Gain/1 -> Sum1/1
  Sum1/1 -> u_ideal/1
  MATLAB Function/1(offA_vec) -> Gain1/1
  Gain1/1 -> Sum1/2

== system SADproject/(De-tumbling + Slew maneuver) Thrusters/Control logic/Subsystem8 ==
  om : Inport
  Dot Product : DotProduct  OutDataTypeStr=Inherit: Inherit via internal rule
  Sqrt : Sqrt
  norm : Outport
  wires:
  Sqrt/1 -> norm/1
  Dot Product/1 -> Sqrt/1
  om/1 -> Dot Product/2, Dot Product/1

== system SADproject/(Trajectory tracking) Inertia Wheels/Thruster desaturation control/Subsystem ==
  T_in : Inport
  Relay : Relay  OnSwitchValue=T  OffSwitchValue=0.8*T  OnOutputValue=T
  Scope{3..6} (4 alike) : Scope
  Sum1 : Sum  Inputs=|+-
  Transfer Fcn : TransferFcn  Denominator=[0.1 1]
  T_out : Outport
  wires:
  Sum1/1 -> Transfer Fcn/1, Scope5/1
  T_in/1 -> Sum1/1, Scope3/1
  Transfer Fcn/1 -> Scope4/1, Relay/1
  Relay/1 -> T_out/1, Sum1/2, Scope6/1

== system SADproject/(Trajectory tracking) Inertia Wheels/Thruster desaturation control/Subsystem1 ==
  T_in : Inport
  Relay : Relay  OnSwitchValue=T  OffSwitchValue=0.8*T  OnOutputValue=T
  Scope{3..6} (4 alike) : Scope
  Sum1 : Sum  Inputs=|+-
  Transfer Fcn : TransferFcn  Denominator=[0.1 1]
  T_out : Outport
  wires:
  Relay/1 -> Scope6/1, Sum1/2, T_out/1
  Transfer Fcn/1 -> Relay/1, Scope4/1
  T_in/1 -> Scope3/1, Sum1/1
  Sum1/1 -> Scope5/1, Transfer Fcn/1

== system SADproject/(Trajectory tracking) Inertia Wheels/Thruster desaturation control/Subsystem2 ==
  T_in : Inport
  Relay : Relay  OnSwitchValue=T  OffSwitchValue=0.8*T  OnOutputValue=T
  Scope{3..6} (4 alike) : Scope
  Sum1 : Sum  Inputs=|+-
  Transfer Fcn : TransferFcn  Denominator=[0.1 1]
  T_out : Outport
  wires:
  Sum1/1 -> Transfer Fcn/1, Scope5/1
  T_in/1 -> Sum1/1, Scope3/1
  Transfer Fcn/1 -> Scope4/1, Relay/1
  Relay/1 -> T_out/1, Sum1/2, Scope6/1

== system SADproject/(Trajectory tracking) Inertia Wheels/Thruster desaturation control/Subsystem3 ==
  T_in : Inport
  Relay : Relay  OnSwitchValue=T  OffSwitchValue=0.8*T  OnOutputValue=T
  Scope{3..6} (4 alike) : Scope
  Sum1 : Sum  Inputs=|+-
  Transfer Fcn : TransferFcn  Denominator=[0.1 1]
  T_out : Outport
  wires:
  Relay/1 -> Scope6/1, Sum1/2, T_out/1
  Transfer Fcn/1 -> Relay/1, Scope4/1
  T_in/1 -> Scope3/1, Sum1/1
  Sum1/1 -> Scope5/1, Transfer Fcn/1

== system SADproject/(Trajectory tracking) Inertia Wheels/Thruster desaturation control/Subsystem4 ==
  T_in : Inport
  Relay : Relay  OnSwitchValue=T  OffSwitchValue=0.8*T  OnOutputValue=T
  Scope{3..6} (4 alike) : Scope
  Sum1 : Sum  Inputs=|+-
  Transfer Fcn : TransferFcn  Denominator=[0.1 1]
  T_out : Outport
  wires:
  Sum1/1 -> Transfer Fcn/1, Scope5/1
  T_in/1 -> Sum1/1, Scope3/1
  Transfer Fcn/1 -> Scope4/1, Relay/1
  Relay/1 -> T_out/1, Sum1/2, Scope6/1

== system SADproject/(Trajectory tracking) Inertia Wheels/Thruster desaturation control/Subsystem5 ==
  T_in : Inport
  Relay : Relay  OnSwitchValue=T  OffSwitchValue=0.8*T  OnOutputValue=T
  Scope{3..6} (4 alike) : Scope
  Sum1 : Sum  Inputs=|+-
  Transfer Fcn : TransferFcn  Denominator=[0.1 1]
  T_out : Outport
  wires:
  Relay/1 -> Scope6/1, Sum1/2, T_out/1
  Transfer Fcn/1 -> Relay/1, Scope4/1
  T_in/1 -> Scope3/1, Sum1/1
  Sum1/1 -> Scope5/1, Transfer Fcn/1

== system SADproject/(Trajectory tracking) Inertia Wheels/Thruster desaturation control/Subsystem6 ==
  T_in : Inport
  Relay : Relay  OnSwitchValue=T  OffSwitchValue=0.8*T  OnOutputValue=T
  Scope{3..6} (4 alike) : Scope
  Sum1 : Sum  Inputs=|+-
  Transfer Fcn : TransferFcn  Denominator=[0.1 1]
  T_out : Outport
  wires:
  Sum1/1 -> Transfer Fcn/1, Scope5/1
  T_in/1 -> Sum1/1, Scope3/1
  Transfer Fcn/1 -> Scope4/1, Relay/1
  Relay/1 -> T_out/1, Sum1/2, Scope6/1

== system SADproject/(Trajectory tracking) Inertia Wheels/Thruster desaturation control/Subsystem7 ==
  T_in : Inport
  Relay : Relay  OnSwitchValue=T  OffSwitchValue=0.8*T  OnOutputValue=T
  Scope{3..6} (4 alike) : Scope
  Sum1 : Sum  Inputs=|+-
  Transfer Fcn : TransferFcn  Denominator=[0.1 1]
  T_out : Outport
  wires:
  Relay/1 -> Scope6/1, Sum1/2, T_out/1
  Transfer Fcn/1 -> Relay/1, Scope4/1
  T_in/1 -> Scope3/1, Sum1/1
  Sum1/1 -> Scope5/1, Transfer Fcn/1

== system SADproject/Attitude determination/Attitude errors/Measured ==
  om : Inport
  A_BL* : Inport  Port=2
  MATLAB Function2 : MATLAB Function  TreatAsAtomicUnit=on
  Matrix Multiply1 : Product  Multiplication=Matrix(*)
  Radians to Degrees : simulink_extras/Transformations/Radians to Degrees
  Sum : Sum  Inputs=|+-
  om_L : Constant  Value=[0 0 n]'
  alphas* : Outport
  om_BL* : Outport  Port=2
  wires:
  Radians to Degrees/1 -> alphas*/1
  Matrix Multiply1/1 -> Sum/2
  om_L/1 -> Matrix Multiply1/2
  Sum/1 -> om_BL*/1
  MATLAB Function2/1(y) -> Radians to Degrees/1
  om/1 -> Sum/1
  A_BL*/1 -> MATLAB Function2/1(A), Matrix Multiply1/1

== system SADproject/Attitude determination/Attitude errors/True ==
  A_BL : Inport
  om : Inport  Port=2
  MATLAB Function2 : MATLAB Function  TreatAsAtomicUnit=on
  Matrix Multiply1 : Product  Multiplication=Matrix(*)
  Radians to Degrees : simulink_extras/Transformations/Radians to Degrees
  Sum : Sum  Inputs=|+-
  om_L : Constant  Value=[0 0 n]'
  alphas : Outport
  om_BL : Outport  Port=2
  wires:
  om/1 -> Sum/1
  om_L/1 -> Matrix Multiply1/2
  Matrix Multiply1/1 -> Sum/2
  Sum/1 -> om_BL/1
  A_BL/1 -> MATLAB Function2/1(A), Matrix Multiply1/1
  MATLAB Function2/1(y) -> Radians to Degrees/1
  Radians to Degrees/1 -> alphas/1

== system SADproject/Attitude determination/Gyroscopes/Noise ==
  ARW : RandomNumber  Mean=[0; 0; 0]  Variance=((deg2rad(ARW_gyro))^2)*[1; 1; 1]  Seed=randi(1000, [3, 1])  SampleTime=0.5
  F_gyro : Constant  Value=2000
  Gain2 : Gain  Gain=1/3600
  Product : Product
  Sqrt : Sqrt
  Out1 : Outport
  wires:
  ARW/1 -> Gain2/1  "deg/sqrt(h)"
  Product/1 -> Out1/1
  Sqrt/1 -> Product/2
  F_gyro/1 -> Sqrt/1  "T in h"
  Gain2/1 -> Product/1

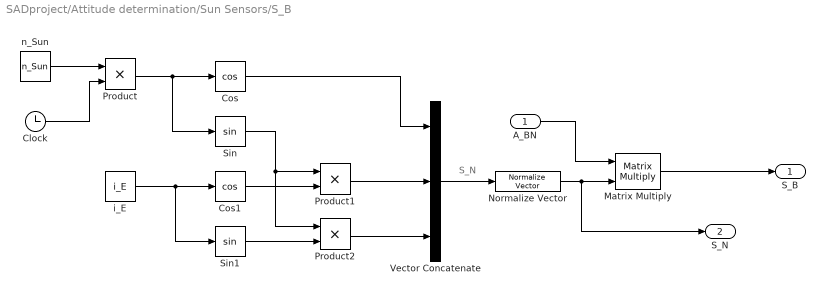
== system SADproject/Attitude determination/Sun Sensors/S_B ==
  note: S_N
  A_BN : Inport
  Clock : Clock
  Cos : Trigonometry  Operator=cos
  Cos1 : Trigonometry  Operator=cos
  Matrix Multiply : Product  Multiplication=Matrix(*)
  Normalize Vector : vrlib/Utilities/Normalize Vector  maxzero=0
  Product : Product
  Product1 : Product
  Product2 : Product
  Sin : Trigonometry
  Sin1 : Trigonometry
  Vector Concatenate : Concatenate  NumInputs=3
  i_E : Constant  Value=i_E
  n_Sun : Constant  Value=n_Sun
  S_B : Outport
  S_N : Outport  Port=2
  wires:
  i_E/1 -> Sin1/1, Cos1/1
  Sin/1 -> Product2/1, Product1/1
  n_Sun/1 -> Product/1
  A_BN/1 -> Matrix Multiply/1
  Vector Concatenate/1 -> Normalize Vector/1
  Product1/1 -> Vector Concatenate/2
  Sin1/1 -> Product2/2
  Product/1 -> Sin/1, Cos/1
  Cos1/1 -> Product1/2
  Product2/1 -> Vector Concatenate/3
  Matrix Multiply/1 -> S_B/1
  Cos/1 -> Vector Concatenate/1
  Normalize Vector/1 -> S_N/1, Matrix Multiply/2
  Clock/1 -> Product/2

== system SADproject/Disturbing Torques/Magnetic perturbation/m_hat ==
  Clock : Clock
  Constant2 : Constant  Value=i_m
  Constant3 : Constant  Value=om_E
  Cos1 : Trigonometry  Operator=cos
  Cos2 : Trigonometry  Operator=cos
  Product : Product
  Product1 : Product
  Product2 : Product
  Scope : Scope
  Sin : Trigonometry
  Sin1 : Trigonometry
  Vector Concatenate : Concatenate  NumInputs=3
  m_hat : Outport
  wires:
  Product2/1 -> Sin1/1, Cos1/1
  Constant3/1 -> Product2/1
  Cos1/1 -> Product/2
  Vector Concatenate/1 -> m_hat/1, Scope/1
  Clock/1 -> Product2/2
  Product/1 -> Vector Concatenate/1
  Constant2/1 -> Sin/1, Cos2/1
  Product1/1 -> Vector Concatenate/2
  Sin/1 -> Product1/1, Product/1
  Cos2/1 -> Vector Concatenate/3
  Sin1/1 -> Product1/2

== system SADproject/Disturbing Torques/SRP perturbation/Direct Solar Radiaton ==
  note: S_B
  A_BN : Inport
  Constant : Constant  Value=N_Bi
  Constant1 : Constant  Value=Ai
  Constant2 : Constant  Value=Ri
  Fe_Sun : Constant  Value=Fe_Sun
  MATLAB Function : MATLAB Function  TreatAsAtomicUnit=on
  S_B : Subsystem
  Scope : Scope
  Transpose : Math  Operator=transpose
  Transpose1 : Math  Operator=transpose
  T_SRP0 : Outport
  wires:
  Fe_Sun/1 -> MATLAB Function/5(Fe)
  Constant1/1 -> MATLAB Function/3(Ai)
  Transpose/1 -> MATLAB Function/1(S_B)
  Constant/1 -> MATLAB Function/2(N_Bi)
  Constant2/1 -> MATLAB Function/4(Ri)
  MATLAB Function/1(T) -> Transpose1/1
  A_BN/1 -> S_B/1(A_BN)
  Transpose1/1 -> T_SRP0/1, Scope/1
  S_B/1(S_B) -> Transpose/1

== system SADproject/Disturbing Torques/SRP perturbation/Earth Radiation ==
  r_B : Inport
  Constant : Constant  Value=N_Bi
  Constant1 : Constant  Value=Ai
  Constant2 : Constant  Value=Ri
  Fe_E : Constant  Value=Fe_E
  MATLAB Function : MATLAB Function  TreatAsAtomicUnit=on
  Scope : Scope
  Transpose : Math  Operator=transpose
  Transpose1 : Math  Operator=transpose
  T_SRP1 : Outport
  wires:
  Transpose1/1 -> T_SRP1/1, Scope/1
  r_B/1 -> Transpose/1
  Constant/1 -> MATLAB Function/2(N_Bi)
  Fe_E/1 -> MATLAB Function/5(Fe)
  Constant2/1 -> MATLAB Function/4(Ri)
  MATLAB Function/1(T) -> Transpose1/1
  Constant1/1 -> MATLAB Function/3(Ai)
  Transpose/1 -> MATLAB Function/1(S_B)

== system SADproject/Disturbing Torques/SRP perturbation/Reflected Radiation ==
  r_B : Inport
  Constant : Constant  Value=N_Bi
  Constant1 : Constant  Value=Ai
  Constant2 : Constant  Value=Ri
  Fe_reflected : Constant  Value=Fe_reflected
  MATLAB Function : MATLAB Function  TreatAsAtomicUnit=on
  Scope : Scope
  Transpose : Math  Operator=transpose
  Transpose1 : Math  Operator=transpose
  T_SRP2 : Outport
  wires:
  MATLAB Function/1(T) -> Transpose1/1
  Constant/1 -> MATLAB Function/2(N_Bi)
  Constant2/1 -> MATLAB Function/4(Ri)
  Constant1/1 -> MATLAB Function/3(Ai)
  Transpose1/1 -> T_SRP2/1, Scope/1
  r_B/1 -> Transpose/1
  Fe_reflected/1 -> MATLAB Function/5(Fe)
  Transpose/1 -> MATLAB Function/1(S_B)

== system SADproject/Orbit model /DCM/Orthonormalization ==
  In1 : Inport
  Gain4 : Gain  Gain=3/2
  Gain5 : Gain  Gain=1/2
  Matri xMultiply2 : Product  Multiplication=Matrix(*)
  MatrixMultiply1 : Product  Multiplication=Matrix(*)
  Sum : Sum  Inputs=|+-
  Transpose : Math  Operator=transpose
  Out1 : Outport
  wires:
  Matri xMultiply2/1 -> Sum/2
  MatrixMultiply1/1 -> Matri xMultiply2/1
  In1/1 -> Gain5/1, Transpose/1, MatrixMultiply1/1, Gain4/1
  Gain4/1 -> Sum/1
  Gain5/1 -> Matri xMultiply2/2
  Transpose/1 -> MatrixMultiply1/2
  Sum/1 -> Out1/1

== system SADproject/Orbit model /DCM/om^ ==
  In1 : Inport
  Gain : Gain  Gain=-1
  Ground : Ground
  Matrix Concatenate : Concatenate  NumInputs=3  Mode=Multidimensional array  ConcatenateDimension=2
  Selector : Selector  InputPortWidth=7  IndexOptions=Index vector (dialog)  Indices=[4 3 6]  OutputSizes=1
  Selector1 : Selector  InputPortWidth=7  IndexOptions=Index vector (dialog)  Indices=[7 4 1]  OutputSizes=1
  Selector2 : Selector  InputPortWidth=7  IndexOptions=Index vector (dialog)  Indices=[2 5 4 ]  OutputSizes=1
  Vector Concatenate : Concatenate  NumInputs=3
  Out1 : Outport
  wires:
  Matrix Concatenate/1 -> Out1/1
  Vector Concatenate/1 -> Selector/1, Selector2/1, Selector1/1
  Ground/1 -> Vector Concatenate/2
  Gain/1 -> Vector Concatenate/3
  In1/1 -> Gain/1, Vector Concatenate/1
  Selector1/1 -> Matrix Concatenate/2
  Selector2/1 -> Matrix Concatenate/3
  Selector/1 -> Matrix Concatenate/1

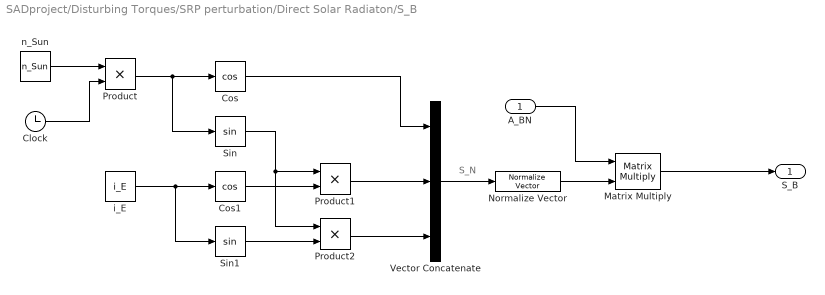
== system SADproject/Disturbing Torques/SRP perturbation/Direct Solar Radiaton/S_B ==
  note: S_N
  A_BN : Inport
  Clock : Clock
  Cos : Trigonometry  Operator=cos
  Cos1 : Trigonometry  Operator=cos
  Matrix Multiply : Product  Multiplication=Matrix(*)
  Normalize Vector : vrlib/Utilities/Normalize Vector  maxzero=0
  Product : Product
  Product1 : Product
  Product2 : Product
  Sin : Trigonometry
  Sin1 : Trigonometry
  Vector Concatenate : Concatenate  NumInputs=3
  i_E : Constant  Value=i_E
  n_Sun : Constant  Value=n_Sun
  S_B : Outport
  wires:
  i_E/1 -> Sin1/1, Cos1/1
  Sin/1 -> Product2/1, Product1/1
  n_Sun/1 -> Product/1
  A_BN/1 -> Matrix Multiply/1
  Vector Concatenate/1 -> Normalize Vector/1
  Product1/1 -> Vector Concatenate/2
  Sin1/1 -> Product2/2
  Product/1 -> Sin/1, Cos/1
  Cos1/1 -> Product1/2
  Product2/1 -> Vector Concatenate/3
  Matrix Multiply/1 -> S_B/1
  Cos/1 -> Vector Concatenate/1
  Normalize Vector/1 -> Matrix Multiply/2
  Clock/1 -> Product/2

== matlab function SADproject/Disturbing Torques/SRP perturbation/Earth Radiation/MATLAB Function ==
  data: S_B input; T output; N_Bi input; Ai input; Ri input; Fe input
function T = SRPtorque(S_B, N_Bi, Ai ,Ri ,Fe)

c  = 2.998*1e8;     % [m/s^2]

P = Fe/c;

rhoS = 0.5;
rhoD = 0.1;

n = length(N_Bi(:,1));

T = [0 0 0];

for i = 1:n
    
    if dot(S_B,N_Bi(i,:)) > 0

        if i>6
            rhoS = 0.1;
        end

        Fi = -P*Ai(i)*dot(S_B,N_Bi(i,:))*((1-rhoS)*S_B+(2*rhoS*dot(S_B,N_Bi(i,:))+2/3*rhoD)*N_Bi(i,:));
        T = T +cross(Ri(i,:),Fi);

    end
end

end

== matlab function SADproject/Disturbing Torques/SRP perturbation/Direct Solar Radiaton/MATLAB Function ==
  data: S_B input; T output; N_Bi input; Ai input; Ri input; Fe input
function T = SRPtorque(S_B, N_Bi, Ai ,Ri ,Fe)

c  = 2.998*1e8;     % [m/s^2]

P = Fe/c;

rhoS = 0.5;
rhoD = 0.1;

n = length(N_Bi(:,1));

T = [0 0 0];

for i = 1:n
    
    if dot(S_B,N_Bi(i,:)) > 0

        if i>6
            rhoS = 0.1;
        end

        Fi = -P*Ai(i)*dot(S_B,N_Bi(i,:))*((1-rhoS)*S_B+(2*rhoS*dot(S_B,N_Bi(i,:))+2/3*rhoD)*N_Bi(i,:));
        T = T +cross(Ri(i,:),Fi);

    end
end

end

== matlab function SADproject/Disturbing Torques/SRP perturbation/Reflected Radiation/MATLAB Function ==
  data: S_B input; T output; N_Bi input; Ai input; Ri input; Fe input
function T = SRPtorque(S_B, N_Bi, Ai ,Ri ,Fe)

c  = 2.998*1e8;     % [m/s^2]

P = Fe/c;

rhoS = 0.5;
rhoD = 0.1;

n = length(N_Bi(:,1));

T = [0 0 0];

for i = 1:n
    
    if dot(S_B,N_Bi(i,:)) > 0

        if i>6
            rhoS = 0.1;
        end

        Fi = -P*Ai(i)*dot(S_B,N_Bi(i,:))*((1-rhoS)*S_B+(2*rhoS*dot(S_B,N_Bi(i,:))+2/3*rhoD)*N_Bi(i,:));
        T = T +cross(Ri(i,:),Fi);

    end
end

end

== matlab function SADproject/(De-tumbling + Slew maneuver) Thrusters/Control logic/Slew maneuver/MATLAB Function ==
  data: A input; offA_vec output
function offA_vec = fcn(A)

offA_vec = [-A(2,3) A(1,3) -A(1,2)]';

end

== matlab function SADproject/Attitude determination/Attitude errors/True/MATLAB Function2 ==
  data: A input; y output
function y = alphas(A)
 
y = [A(2,3) -A(1,3) A(1,2)]';

end

== matlab function SADproject/Attitude determination/Attitude errors/Measured/MATLAB Function2 ==
  data: A input; y output
function y = alphas(A)
 
y = [A(2,3) -A(1,3) A(1,2)]';

end

== matlab function SADproject/State obserever + Linear control/MATLAB Function2 ==
  data: A input; y output
function y = alphas(A)
 
y = [A(2,3) -A(1,3) A(1,2)]';

end
